simulink library "TYPEC_SINGLE_MASTER"  (Simulink 8.8)
settings: Solver=ode45  StartTime=0.0  StopTime=10.0  RelTol=1e-3  EnableMultiTasking=on
libraries: cdsEpicsIn x10, cdsEpicsStringIn x6, cdsEpicsBinIn x4, cdsFilt x4, STATE_BIO_MASTER x2, cdsDacKill x2, cdsEpicsOut x2, VIS_LIB x2, ISC_common x2, SINGLE_OPLEV_NOOSEM_MASTER x2, cdsEpicsMomentary x2
settings Model: SuppressorTable=22 serialization::archive 11 0 3 0 0 0 11 0  Creator=controls  LastModifiedBy=controls

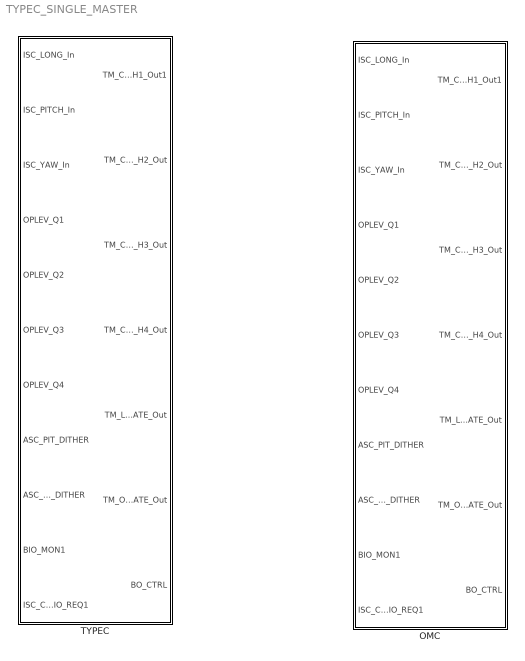
== system TYPEC_SINGLE_MASTER ==
  OMC : Subsystem  Description=TYPEC SINGLE MASTER
      settings: AttributesFormatString=%<Description>
  TYPEC : Subsystem  Description=TYPEC SINGLE MASTER
      settings: AttributesFormatString=%<Description>

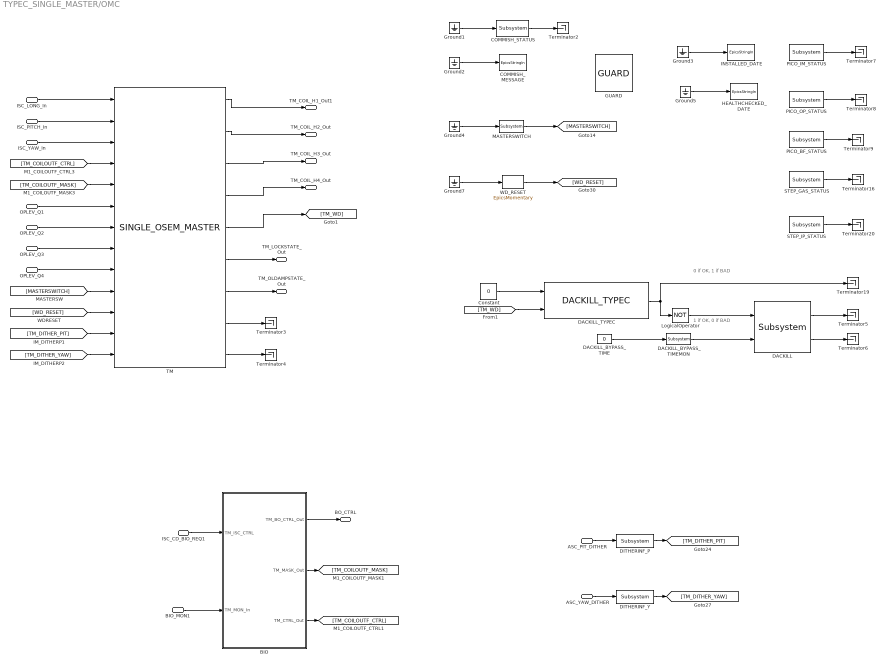
== system TYPEC_SINGLE_MASTER/OMC ==
  note: 0 if OK, 1 if BAD
  note: 1 if OK, 0 if BAD
  ISC_LONG_In : Inport
  ISC_PITCH_In : Inport  Port=2
  ISC_YAW_In : Inport  Port=3
  OPLEV_Q1 : Inport  Port=4
  OPLEV_Q2 : Inport  Port=5
  OPLEV_Q3 : Inport  Port=6
  OPLEV_Q4 : Inport  Port=7
  ASC_PIT_DITHER : Inport  Port=8
  ASC_YAW_DITHER : Inport  Port=9
  BIO_MON1 : Inport  Port=10
  ISC_CD_BIO_REQ1 : Inport  Port=11
  BIO : Subsystem
  COMMISH_MESSAGE : cdsEpicsStringIn/EpicsStringIn  Tag=cdsEpicsStringIn  Description=cdsEpicsStringIn
      settings: AttributesFormatString=%<Tag>
  COMMISH_STATUS : cdsEpicsBinIn/Subsystem  Tag=cdsEpicsBinIn  Description=|
      | Purpose:                                                                            
      | Create an EPICS binary (0 or 1) input channel to the FE realtime controls.          
      |                                                                                     
      | Operation:                                                                          
      | Outputs value from an EPICS ai record. Value is binary input (bi Epics record type).
      |                                                                                     
      | Usage:                                                                              
      | Name the part with the desired EPICS channel name.
      settings: AttributesFormatString=%<Tag>
  Constant : Constant  Value=0
  DACKILL : cdsDacKill/Subsystem  Description=cdsDacKill
      settings: AttributesFormatString=%<Description>
  DACKILL_BYPASS_TIME : Constant  Value=0
  DACKILL_BYPASS_TIMEMON : cdsEpicsOut/Subsystem  Tag=cdsEpicsOutput  Description=|
      | Purpose:                                          
      | Output a FE signal to an EPICS channel.           
      |                                                   
      | Operation:                                        
      | Takes input value and passes it to EPICS record.  
      |                                                   
      | Usage:                                            
      | Name the part with the desired EPICS rrecord name.
      settings: AttributesFormatString=%<Tag>
  DACKILL_TYPEC : VIS_LIB/DACKILL_TYPEC 
  DITHERINF_P : cdsFilt/Subsystem  Tag=cdsFilt  Description=|
      | Purpose:                                                                                                                                                                                                                                  
      | Standard CDS IIR filter module.                                                                                                                                                                                                           
      |                                                                                                                                                                                                                                           
      | Operation:                                                                                                                                                                                                                                
      | Consists of 10 second order section IIR filters, plus a ramped gain stage. In FE code, also provides pre-defined test points and excitation channel inputs. The filter coefficients are defined in the LIGO system using the 'foton' tool.
      |                                                                                                                                                                                                                                           
      | Usage:                                                                                                                                                                                                                                    
      | Name the part with the desired filter module name.
      settings: AttributesFormatString=%<Tag>
  DITHERINF_Y : cdsFilt/Subsystem  Tag=cdsFilt  Description=|
      | Purpose:                                                                                                                                                                                                                                  
      | Standard CDS IIR filter module.                                                                                                                                                                                                           
      |                                                                                                                                                                                                                                           
      | Operation:                                                                                                                                                                                                                                
      | Consists of 10 second order section IIR filters, plus a ramped gain stage. In FE code, also provides pre-defined test points and excitation channel inputs. The filter coefficients are defined in the LIGO system using the 'foton' tool.
      |                                                                                                                                                                                                                                           
      | Usage:                                                                                                                                                                                                                                    
      | Name the part with the desired filter module name.
      settings: AttributesFormatString=%<Tag>
  GUARD : ISC_common/GUARD
  Ground{1..5,7} (6 alike) : Ground
  HEALTHCHECKED_DATE : cdsEpicsStringIn/EpicsStringIn  Tag=cdsEpicsStringIn  Description=cdsEpicsStringIn
      settings: AttributesFormatString=%<Tag>
  INSTALLED_DATE : cdsEpicsStringIn/EpicsStringIn  Tag=cdsEpicsStringIn  Description=cdsEpicsStringIn
      settings: AttributesFormatString=%<Tag>
  LogicalOperator : Logic  Operator=NOT  AllPortsSameDT=off  OutDataTypeStr=boolean
  MASTERSWITCH : cdsEpicsBinIn/Subsystem  Tag=cdsEpicsBinIn  Description=|
      | Purpose:                                                                            
      | Create an EPICS binary (0 or 1) input channel to the FE realtime controls.          
      |                                                                                     
      | Operation:                                                                          
      | Outputs value from an EPICS ai record. Value is binary input (bi Epics record type).
      |                                                                                     
      | Usage:                                                                              
      | Name the part with the desired EPICS channel name.
      settings: AttributesFormatString=%<Tag>
  PICO_BF_STATUS : cdsEpicsIn/Subsystem  Tag=cdsEpicsIn  Description=|
      | Purpose:                                                                              
      | Create an EPICS input channel connection to the FE realtime controls.                 
      |                                                                                       
      | Operation:                                                                            
      | Outputs value from an EPICS ai record. Value is floating point with a precision of 3..
      |                                                                                       
      | Usage:                                                                                
      | Name the part with the desired EPICS channel name.
      settings: AttributesFormatString=%<Tag>
  PICO_IM_STATUS : cdsEpicsIn/Subsystem  Tag=cdsEpicsIn  Description=|
      | Purpose:                                                                              
      | Create an EPICS input channel connection to the FE realtime controls.                 
      |                                                                                       
      | Operation:                                                                            
      | Outputs value from an EPICS ai record. Value is floating point with a precision of 3..
      |                                                                                       
      | Usage:                                                                                
      | Name the part with the desired EPICS channel name.
      settings: AttributesFormatString=%<Tag>
  PICO_OP_STATUS : cdsEpicsIn/Subsystem  Tag=cdsEpicsIn  Description=|
      | Purpose:                                                                              
      | Create an EPICS input channel connection to the FE realtime controls.                 
      |                                                                                       
      | Operation:                                                                            
      | Outputs value from an EPICS ai record. Value is floating point with a precision of 3..
      |                                                                                       
      | Usage:                                                                                
      | Name the part with the desired EPICS channel name.
      settings: AttributesFormatString=%<Tag>
  STEP_GAS_STATUS : cdsEpicsIn/Subsystem  Tag=cdsEpicsIn  Description=|
      | Purpose:                                                                              
      | Create an EPICS input channel connection to the FE realtime controls.                 
      |                                                                                       
      | Operation:                                                                            
      | Outputs value from an EPICS ai record. Value is floating point with a precision of 3..
      |                                                                                       
      | Usage:                                                                                
      | Name the part with the desired EPICS channel name.
      settings: AttributesFormatString=%<Tag>
  STEP_IP_STATUS : cdsEpicsIn/Subsystem  Tag=cdsEpicsIn  Description=|
      | Purpose:                                                                              
      | Create an EPICS input channel connection to the FE realtime controls.                 
      |                                                                                       
      | Operation:                                                                            
      | Outputs value from an EPICS ai record. Value is floating point with a precision of 3..
      |                                                                                       
      | Usage:                                                                                
      | Name the part with the desired EPICS channel name.
      settings: AttributesFormatString=%<Tag>
  TM : SINGLE_OPLEV_NOOSEM_MASTER/SINGLE_OSEM_MASTER
  Terminator{2..9,16,19..20} (11 alike) : Terminator
  WD_RESET : cdsEpicsMomentary/EpicsMomentary  Tag=cdsEpicsMomentary
      settings: AttributesFormatString=%<Tag>
  TM_COIL_H1_Out1 : Outport
  TM_COIL_H2_Out : Outport  Port=2
  TM_COIL_H3_Out : Outport  Port=3
  TM_COIL_H4_Out : Outport  Port=4
  TM_LOCKSTATE_Out : Outport  Port=5
  TM_OLDAMPSTATE_Out : Outport  Port=6
  BO_CTRL : Outport  Port=7
  wires:
  TM/9 -> Terminator4/1
  TM/2 -> TM_COIL_H2_Out/1
  TM/1 -> TM_COIL_H1_Out1/1
  TM/4 -> TM_COIL_H4_Out/1
  TM/3 -> TM_COIL_H3_Out/1
  [TM_WD] -> DACKILL_TYPEC/2
  Constant/1 -> DACKILL_TYPEC/1
  DACKILL_TYPEC/1 -> Terminator19/1, LogicalOperator/1
  LogicalOperator/1 -> DACKILL/1
  DACKILL_BYPASS_TIMEMON/1 -> DACKILL/2
  DACKILL_BYPASS_TIME/1 -> DACKILL_BYPASS_TIMEMON/1
  DACKILL/1 -> Terminator5/1
  DACKILL/2 -> Terminator6/1
  [TM_DITHER_YAW] -> TM/13
  [TM_DITHER_PIT] -> TM/12
  DITHERINF_Y/1 -> [TM_DITHER_YAW]
  DITHERINF_P/1 -> [TM_DITHER_PIT]
  ASC_PIT_DITHER/1 -> DITHERINF_P/1
  ASC_YAW_DITHER/1 -> DITHERINF_Y/1
  Ground1/1 -> COMMISH_STATUS/1
  COMMISH_STATUS/1 -> Terminator2/1
  Ground2/1 -> COMMISH_MESSAGE/1
  ISC_LONG_In/1 -> TM/1
  TM/5 -> [TM_WD]
  MASTERSWITCH/1 -> [MASTERSWITCH]
  Ground4/1 -> MASTERSWITCH/1
  OPLEV_Q1/1 -> TM/6
  OPLEV_Q2/1 -> TM/7
  OPLEV_Q3/1 -> TM/8
  ISC_PITCH_In/1 -> TM/2
  ISC_YAW_In/1 -> TM/3
  OPLEV_Q4/1 -> TM/9
  [MASTERSWITCH] -> TM/10
  Ground7/1 -> WD_RESET/1
  WD_RESET/1 -> [WD_RESET]
  [WD_RESET] -> TM/11
  BIO_MON1/1 -> BIO/2(TM_MON_In)
  ISC_CD_BIO_REQ1/1 -> BIO/1(TM_ISC_CTRL)
  BIO/2(TM_MASK_Out) -> [TM_COILOUTF_MASK]
  BIO/3(TM_CTRL_Out) -> [TM_COILOUTF_CTRL]
  [TM_COILOUTF_CTRL] -> TM/4
  [TM_COILOUTF_MASK] -> TM/5
  BIO/1(TM_BO_CTRL_Out) -> BO_CTRL/1
  TM/6 -> TM_LOCKSTATE_Out/1
  TM/7 -> TM_OLDAMPSTATE_Out/1
  TM/8 -> Terminator3/1
  Ground3/1 -> INSTALLED_DATE/1
  Ground5/1 -> HEALTHCHECKED_DATE/1
  STEP_IP_STATUS/1 -> Terminator20/1
  STEP_GAS_STATUS/1 -> Terminator16/1
  PICO_BF_STATUS/1 -> Terminator9/1
  PICO_IM_STATUS/1 -> Terminator7/1
  PICO_OP_STATUS/1 -> Terminator8/1

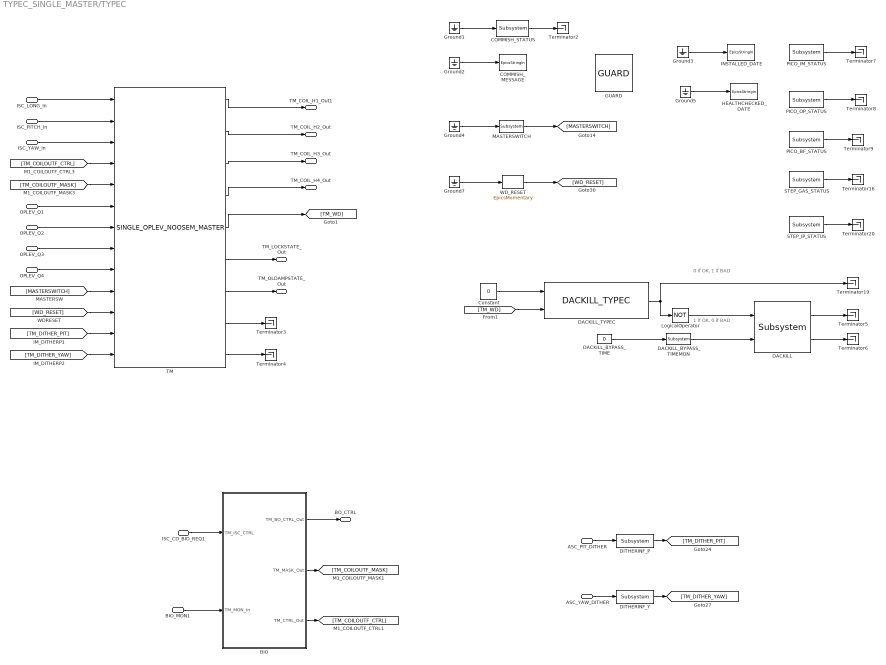
== system TYPEC_SINGLE_MASTER/TYPEC ==
  note: 0 if OK, 1 if BAD
  note: 1 if OK, 0 if BAD
  ISC_LONG_In : Inport
  ISC_PITCH_In : Inport  Port=2
  ISC_YAW_In : Inport  Port=3
  OPLEV_Q1 : Inport  Port=4
  OPLEV_Q2 : Inport  Port=5
  OPLEV_Q3 : Inport  Port=6
  OPLEV_Q4 : Inport  Port=7
  ASC_PIT_DITHER : Inport  Port=8
  ASC_YAW_DITHER : Inport  Port=9
  BIO_MON1 : Inport  Port=10
  ISC_CD_BIO_REQ1 : Inport  Port=11
  BIO : Subsystem
  COMMISH_MESSAGE : cdsEpicsStringIn/EpicsStringIn  Tag=cdsEpicsStringIn  Description=cdsEpicsStringIn
      settings: AttributesFormatString=%<Tag>
  COMMISH_STATUS : cdsEpicsBinIn/Subsystem  Tag=cdsEpicsBinIn  Description=|
      | Purpose:                                                                            
      | Create an EPICS binary (0 or 1) input channel to the FE realtime controls.          
      |                                                                                     
      | Operation:                                                                          
      | Outputs value from an EPICS ai record. Value is binary input (bi Epics record type).
      |                                                                                     
      | Usage:                                                                              
      | Name the part with the desired EPICS channel name.
      settings: AttributesFormatString=%<Tag>
  Constant : Constant  Value=0
  DACKILL : cdsDacKill/Subsystem  Description=cdsDacKill
      settings: AttributesFormatString=%<Description>
  DACKILL_BYPASS_TIME : Constant  Value=0
  DACKILL_BYPASS_TIMEMON : cdsEpicsOut/Subsystem  Tag=cdsEpicsOutput  Description=|
      | Purpose:                                          
      | Output a FE signal to an EPICS channel.           
      |                                                   
      | Operation:                                        
      | Takes input value and passes it to EPICS record.  
      |                                                   
      | Usage:                                            
      | Name the part with the desired EPICS rrecord name.
      settings: AttributesFormatString=%<Tag>
  DACKILL_TYPEC : VIS_LIB/DACKILL_TYPEC 
  DITHERINF_P : cdsFilt/Subsystem  Tag=cdsFilt  Description=|
      | Purpose:                                                                                                                                                                                                                                  
      | Standard CDS IIR filter module.                                                                                                                                                                                                           
      |                                                                                                                                                                                                                                           
      | Operation:                                                                                                                                                                                                                                
      | Consists of 10 second order section IIR filters, plus a ramped gain stage. In FE code, also provides pre-defined test points and excitation channel inputs. The filter coefficients are defined in the LIGO system using the 'foton' tool.
      |                                                                                                                                                                                                                                           
      | Usage:                                                                                                                                                                                                                                    
      | Name the part with the desired filter module name.
      settings: AttributesFormatString=%<Tag>
  DITHERINF_Y : cdsFilt/Subsystem  Tag=cdsFilt  Description=|
      | Purpose:                                                                                                                                                                                                                                  
      | Standard CDS IIR filter module.                                                                                                                                                                                                           
      |                                                                                                                                                                                                                                           
      | Operation:                                                                                                                                                                                                                                
      | Consists of 10 second order section IIR filters, plus a ramped gain stage. In FE code, also provides pre-defined test points and excitation channel inputs. The filter coefficients are defined in the LIGO system using the 'foton' tool.
      |                                                                                                                                                                                                                                           
      | Usage:                                                                                                                                                                                                                                    
      | Name the part with the desired filter module name.
      settings: AttributesFormatString=%<Tag>
  GUARD : ISC_common/GUARD
  Ground{1..5,7} (6 alike) : Ground
  HEALTHCHECKED_DATE : cdsEpicsStringIn/EpicsStringIn  Tag=cdsEpicsStringIn  Description=cdsEpicsStringIn
      settings: AttributesFormatString=%<Tag>
  INSTALLED_DATE : cdsEpicsStringIn/EpicsStringIn  Tag=cdsEpicsStringIn  Description=cdsEpicsStringIn
      settings: AttributesFormatString=%<Tag>
  LogicalOperator : Logic  Operator=NOT  AllPortsSameDT=off  OutDataTypeStr=boolean
  MASTERSWITCH : cdsEpicsBinIn/Subsystem  Tag=cdsEpicsBinIn  Description=|
      | Purpose:                                                                            
      | Create an EPICS binary (0 or 1) input channel to the FE realtime controls.          
      |                                                                                     
      | Operation:                                                                          
      | Outputs value from an EPICS ai record. Value is binary input (bi Epics record type).
      |                                                                                     
      | Usage:                                                                              
      | Name the part with the desired EPICS channel name.
      settings: AttributesFormatString=%<Tag>
  PICO_BF_STATUS : cdsEpicsIn/Subsystem  Tag=cdsEpicsIn  Description=|
      | Purpose:                                                                              
      | Create an EPICS input channel connection to the FE realtime controls.                 
      |                                                                                       
      | Operation:                                                                            
      | Outputs value from an EPICS ai record. Value is floating point with a precision of 3..
      |                                                                                       
      | Usage:                                                                                
      | Name the part with the desired EPICS channel name.
      settings: AttributesFormatString=%<Tag>
  PICO_IM_STATUS : cdsEpicsIn/Subsystem  Tag=cdsEpicsIn  Description=|
      | Purpose:                                                                              
      | Create an EPICS input channel connection to the FE realtime controls.                 
      |                                                                                       
      | Operation:                                                                            
      | Outputs value from an EPICS ai record. Value is floating point with a precision of 3..
      |                                                                                       
      | Usage:                                                                                
      | Name the part with the desired EPICS channel name.
      settings: AttributesFormatString=%<Tag>
  PICO_OP_STATUS : cdsEpicsIn/Subsystem  Tag=cdsEpicsIn  Description=|
      | Purpose:                                                                              
      | Create an EPICS input channel connection to the FE realtime controls.                 
      |                                                                                       
      | Operation:                                                                            
      | Outputs value from an EPICS ai record. Value is floating point with a precision of 3..
      |                                                                                       
      | Usage:                                                                                
      | Name the part with the desired EPICS channel name.
      settings: AttributesFormatString=%<Tag>
  STEP_GAS_STATUS : cdsEpicsIn/Subsystem  Tag=cdsEpicsIn  Description=|
      | Purpose:                                                                              
      | Create an EPICS input channel connection to the FE realtime controls.                 
      |                                                                                       
      | Operation:                                                                            
      | Outputs value from an EPICS ai record. Value is floating point with a precision of 3..
      |                                                                                       
      | Usage:                                                                                
      | Name the part with the desired EPICS channel name.
      settings: AttributesFormatString=%<Tag>
  STEP_IP_STATUS : cdsEpicsIn/Subsystem  Tag=cdsEpicsIn  Description=|
      | Purpose:                                                                              
      | Create an EPICS input channel connection to the FE realtime controls.                 
      |                                                                                       
      | Operation:                                                                            
      | Outputs value from an EPICS ai record. Value is floating point with a precision of 3..
      |                                                                                       
      | Usage:                                                                                
      | Name the part with the desired EPICS channel name.
      settings: AttributesFormatString=%<Tag>
  TM : SINGLE_OPLEV_NOOSEM_MASTER/SINGLE_OPLEV_NOOSEM_MASTER
  Terminator{2..9,16,19..20} (11 alike) : Terminator
  WD_RESET : cdsEpicsMomentary/EpicsMomentary  Tag=cdsEpicsMomentary
      settings: AttributesFormatString=%<Tag>
  TM_COIL_H1_Out1 : Outport
  TM_COIL_H2_Out : Outport  Port=2
  TM_COIL_H3_Out : Outport  Port=3
  TM_COIL_H4_Out : Outport  Port=4
  TM_LOCKSTATE_Out : Outport  Port=5
  TM_OLDAMPSTATE_Out : Outport  Port=6
  BO_CTRL : Outport  Port=7
  wires:
  TM/9 -> Terminator4/1
  TM/2 -> TM_COIL_H2_Out/1
  TM/1 -> TM_COIL_H1_Out1/1
  TM/4 -> TM_COIL_H4_Out/1
  TM/3 -> TM_COIL_H3_Out/1
  [TM_WD] -> DACKILL_TYPEC/2
  Constant/1 -> DACKILL_TYPEC/1
  DACKILL_TYPEC/1 -> Terminator19/1, LogicalOperator/1
  LogicalOperator/1 -> DACKILL/1
  DACKILL_BYPASS_TIMEMON/1 -> DACKILL/2
  DACKILL_BYPASS_TIME/1 -> DACKILL_BYPASS_TIMEMON/1
  DACKILL/1 -> Terminator5/1
  DACKILL/2 -> Terminator6/1
  [TM_DITHER_YAW] -> TM/13
  [TM_DITHER_PIT] -> TM/12
  DITHERINF_Y/1 -> [TM_DITHER_YAW]
  DITHERINF_P/1 -> [TM_DITHER_PIT]
  ASC_PIT_DITHER/1 -> DITHERINF_P/1
  ASC_YAW_DITHER/1 -> DITHERINF_Y/1
  Ground1/1 -> COMMISH_STATUS/1
  COMMISH_STATUS/1 -> Terminator2/1
  Ground2/1 -> COMMISH_MESSAGE/1
  ISC_LONG_In/1 -> TM/1
  TM/5 -> [TM_WD]
  MASTERSWITCH/1 -> [MASTERSWITCH]
  Ground4/1 -> MASTERSWITCH/1
  OPLEV_Q1/1 -> TM/6
  OPLEV_Q2/1 -> TM/7
  OPLEV_Q3/1 -> TM/8
  ISC_PITCH_In/1 -> TM/2
  ISC_YAW_In/1 -> TM/3
  OPLEV_Q4/1 -> TM/9
  [MASTERSWITCH] -> TM/10
  Ground7/1 -> WD_RESET/1
  WD_RESET/1 -> [WD_RESET]
  [WD_RESET] -> TM/11
  BIO_MON1/1 -> BIO/2(TM_MON_In)
  ISC_CD_BIO_REQ1/1 -> BIO/1(TM_ISC_CTRL)
  BIO/2(TM_MASK_Out) -> [TM_COILOUTF_MASK]
  BIO/3(TM_CTRL_Out) -> [TM_COILOUTF_CTRL]
  [TM_COILOUTF_CTRL] -> TM/4
  [TM_COILOUTF_MASK] -> TM/5
  BIO/1(TM_BO_CTRL_Out) -> BO_CTRL/1
  TM/6 -> TM_LOCKSTATE_Out/1
  TM/7 -> TM_OLDAMPSTATE_Out/1
  TM/8 -> Terminator3/1
  Ground3/1 -> INSTALLED_DATE/1
  Ground5/1 -> HEALTHCHECKED_DATE/1
  STEP_IP_STATUS/1 -> Terminator20/1
  STEP_GAS_STATUS/1 -> Terminator16/1
  PICO_BF_STATUS/1 -> Terminator9/1
  PICO_IM_STATUS/1 -> Terminator7/1
  PICO_OP_STATUS/1 -> Terminator8/1

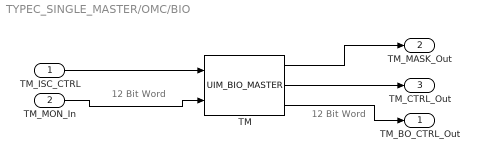
== system TYPEC_SINGLE_MASTER/OMC/BIO ==
  note: 12 Bit Word
  note: 12 Bit Word
  TM_ISC_CTRL : Inport
  TM_MON_In : Inport  Port=2
  TM : STATE_BIO_MASTER/UIM_BIO_MASTER
  TM_BO_CTRL_Out : Outport
  TM_MASK_Out : Outport  Port=2
  TM_CTRL_Out : Outport  Port=3
  wires:
  TM/2 -> TM_CTRL_Out/1
  TM/1 -> TM_MASK_Out/1
  TM/3 -> TM_BO_CTRL_Out/1
  TM_MON_In/1 -> TM/2
  TM_ISC_CTRL/1 -> TM/1

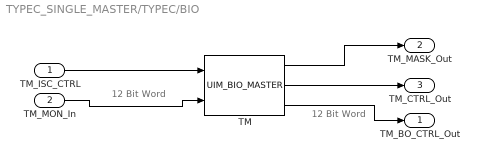
== system TYPEC_SINGLE_MASTER/TYPEC/BIO ==
  note: 12 Bit Word
  note: 12 Bit Word
  TM_ISC_CTRL : Inport
  TM_MON_In : Inport  Port=2
  TM : STATE_BIO_MASTER/UIM_BIO_MASTER
  TM_BO_CTRL_Out : Outport
  TM_MASK_Out : Outport  Port=2
  TM_CTRL_Out : Outport  Port=3
  wires:
  TM/2 -> TM_CTRL_Out/1
  TM/1 -> TM_MASK_Out/1
  TM/3 -> TM_BO_CTRL_Out/1
  TM_MON_In/1 -> TM/2
  TM_ISC_CTRL/1 -> TM/1
